simulink library "sm_backhoe_lib"  (R2021b)
settings: Solver=ode45  StartTime=0.0  StopTime=10.0  RelTol=1e-3  EnableMultiTasking=on
undefined symbols (not defined in the file): X, Y, Z
libraries: sm_lib x45, fl_lib x12, $bdroot x7, nesl_utility x4, simulink x1
(part 1 of 2)
settings Model: Creator=The MathWorks, Inc.  LastModifiedBy=The MathWorks, Inc.
settings SolverCC: AlgebraicLoopSolver=TrustRegion
settings DataIOCC: LimitDataPoints=on  SaveFormat=Array  SignalLoggingSaveFormat=ModelDataLogs  ReturnWorkspaceOutputs=off
settings OptimizationCC: ExpressionDepthLimit=2147483647  LifeSpan=inf
settings DebuggingCC: UnderspecifiedInitializationDetection=Classic  MergeDetectMultiDrivingBlocksExec=none  SolverPrmCheckMsg=warning  MultiTaskDSMMsg=warning  MultiTaskCondExecSysMsg=none  StateNameClashWarn=warning  SFUnexpectedBacktrackingDiag=warning  SFNoUnconditionalDefaultTransitionDiag=warning  SFExecutionAtInitializationDiag=none  SFMachineParentedDataDiag=warning  ArithmeticOperatorsInVariantConditions=warning
settings HardwareCC: ProdBitPerPointer=32  ProdBitPerSizeT=32  ProdBitPerPtrDiffT=32  ProdLargestAtomicFloat=None  ProdIntDivRoundTo=Undefined  ProdEndianess=Unspecified  ProdWordSize=32  ProdHWDeviceType=32-bit Generic
settings ModelReferenceCC: PropagateSignalLabelsOutOfModel=off
settings SFSimCC: SimUseLocalCustomCode=off  CustomCodeUndefinedFunction=UseInterfaceOnly
settings RTWCC: RTWUseLocalCustomCode=off
settings CodeAppCC: StateflowObjectComments=on
settings GRTTargetCC: TargetLangStandard=C89/C90 (ANSI)
settings ConfigComp: CovMetricSettings=dw  CovSaveCumulativeToWorkspaceVar=on  CovSaveSingleToWorkspaceVar=on  CovExternalEMLEnable=off

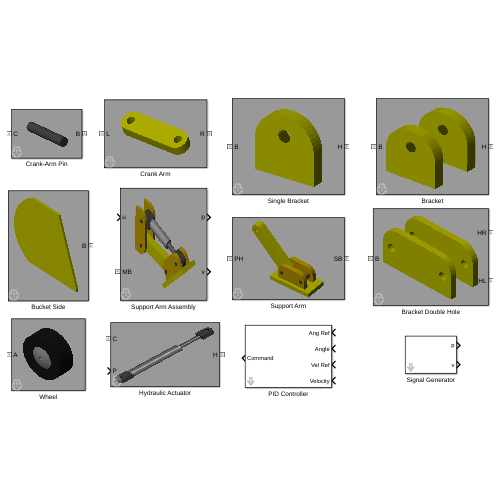
[thumbnail: Simulink's stored preview of the top-level diagram]
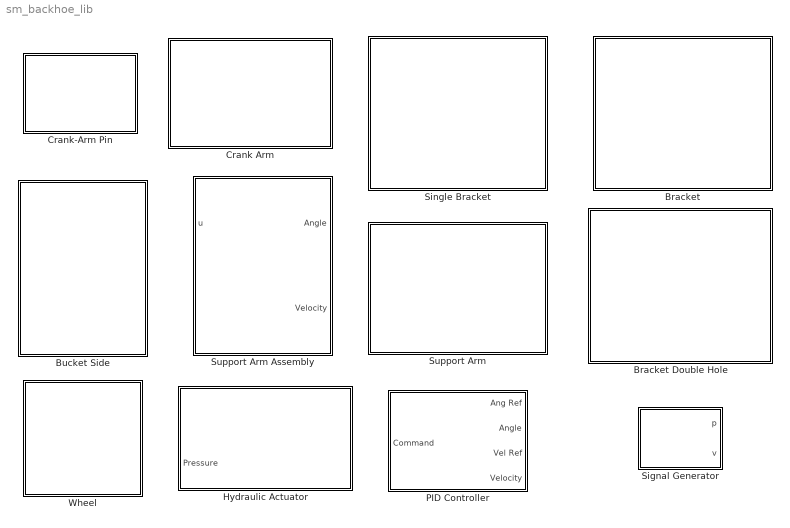
== system sm_backhoe_lib ==
  Bracket : Subsystem  mask(Bracket){Hbracket=0.75, Wbracket=0.75, Tbracket=0.15, Dbracket=0.8, Hhole=0.5, Rhole=0.075, circlePoints=25, bracketColor=[0.8 0.8 0], rho=7780}
      mask prompts: Hbracket "Hbracket (m)"; Wbracket "Wbracket (m)"; Tbracket "Tbracket (m)"; Dbracket "Dbracket (m)"; Hhole "Hhole (m)"; Rhole "Rhole (m)"; circlePoints "Circle Resolution (pts/rev)"; bracketColor "Bracket Color"; rho "Density (kg/m^3)"
      mask help:
      | Consists of the backhoe bracket assembly.
      |
      | Attachment points are:
      | B: The base of the bracket.
      | H: The center point between the two holes, which is configured for Revolute joints.
      |
      | Click on Help to view a schematic of the bracket, its configurable dimension parameters and attachment points (in red).
      mask init:
      | bracketPoints = [];
      | 
      | %% Bracket mold.
      | y = Hbracket - (Wbracket/2);
      | for i = 0:circlePoints
      |     angle = (i/circlePoints)*pi;
      |     bracketPoints = [bracketPoints; ...
      |                     (Wbracket/2)*cos(angle) (y+(Wbracket/2)*sin(angle))];
      | end
      | bracketPoints = [bracketPoints; ...
      |                  -Wbracket/2 0;0 0];
      |              
      | %% Hole
      | for i = 0:circlePoints*2
      |     angle = -pi/2 - (i/circlePoints)*pi;
      |     bracketPoints = [bracketPoints; ...
      |                     Rhole*cos(angle) (Hhole+(Rhole*sin(angle)))];
      | end
      | bracketPoints = [bracketPoints; ...
      |                  0 0;Wbracket/2 0];
      |                  
      | %% Uncomment to plot the cross-sections
      | % close all;
      | % figure;
      | % plot(bracketPoints(:,1),bracketPoints(:,2),'b*-');
      mask Help: web(fullfile(matlabroot,'toolbox','physmod','sm','smdemos','backhoe','demohelp','sm_backhoe_bracket.html'));
      mask Display:
      | image(fullfile(matlabroot,'toolbox','physmod','sm','smdemos','backhoe','images','sm_backhoe_bracket.png'));
      | port_label('lconn',1,'B');
      | port_label('rconn',1,'H');
  Bracket Double Hole : Subsystem  mask(Bracket Double Hole){Hbracket=1, Wbracket=2, Tbracket=0.15, Dbracket=0.8, Hhole=0.5, Dhole=1.5, Rhole=0.1, Rfillet=0.4, Nc=25, bracketColor=[0.8 0.8 0], rho=7780}
      mask prompts: Hbracket "Hbracket (m)"; Wbracket "Wbracket (m)"; Tbracket "Tbracket (m)"; Dbracket "Dbracket (m)"; Hhole "Hhole (m)"; Dhole "Dhole (m)"; Rhole "Rhole (m)"; Rfillet "Rfillet (m)"; Nc "Circle Resolution (pts/rev)"; bracketColor "Bracket Color"; rho "Density (kg/m^3)"
      mask help:
      | Consists of the backhoe double-hole bracket assembly.
      |
      | Attachment points are:
      | B: The base of the bracket.
      | HL: The center point between the two left holes, which is configured for Revolute joints.
      | HR: The center point between the two right holes, which is configured for Revolute joints.
      |
      | Click on Help to view a schematic of the bracket, its configurable dimension parameters and attachment points (in red).
      mask init:
      | %% Right Hole
      | bracketPoints = [0 0; Dhole/2 0];
      | angle = linspace(-pi/2,-5*pi/2,Nc)';
      | bracketPoints = [bracketPoints; ...
      |                  (Dhole/2+Rhole*cos(angle)) (Hhole+Rhole*sin(angle))];
      | bracketPoints = [bracketPoints; Dhole/2 0];                 
      | 
      | %% Bracket Outer Boundary
      | bracketPoints = [bracketPoints; Wbracket/2 0];
      | x = Wbracket/2 - Rfillet;
      | y = Hbracket - Rfillet;
      | angle = linspace(0,pi/2,Nc/4)';
      | bracketPoints = [bracketPoints; ...
      |                  (x+Rfillet*cos(angle)) (y+Rfillet*sin(angle))];
      | 
      | angle = linspace(pi/2,pi,Nc/4)';             
      | bracketPoints = [bracketPoints; ...
      |                  (-x+Rfillet*cos(angle)) (y+Rfillet*sin(angle))];
      | bracketPoints = [bracketPoints; -Wbracket/2 0];
      |                  
      | %% Left Hole
      | bracketPoints = [bracketPoints;-Dhole/2 0];
      | angle = linspace(-pi/2,-5*pi/2,Nc)';
      | bracketPoints = [bracketPoints; ...
      |                  (-Dhole/2+Rhole*cos(angle)) (Hhole+Rhole*sin(angle))];
      | bracketPoints = [bracketPoints;-Dhole/2 0];
      mask Help: web(fullfile(matlabroot,'toolbox','physmod','sm','smdemos','backhoe','demohelp','sm_backhoe_bracket2.html'));
      mask Display:
      | image(fullfile(matlabroot,'toolbox','physmod','sm','smdemos','backhoe','images','sm_backhoe_bracket2.png'));
      | port_label('lconn',1,'B');
      | port_label('rconn',1,'HR');
      | port_label('rconn',2,'HL');
  Bucket Side : Subsystem  mask(Bucket Side){bucketUpper=1.3, bucketLower=2, bucketHeight=2, bucketThickness=0.05, chordAngle=pi/6, Nc=45, color=[0.8 0.8 0], rho=7780}
      mask prompts: bucketUpper "Wupper (m)"; bucketLower "Wlower (m)"; bucketHeight "Hbucket (m)"; bucketThickness "Tbucket (m)"; chordAngle "alpha (radians)"; Nc "Circle Resolution (pts/rev)"; rho "Density (kg/m^3)"
      mask help:
      | Consists of the backhoe bucket side plate, which is used as an auxiliary library block inside the Bucket block.
      |
      | Click on Help to view a schematic of the bucket, its configurable dimension parameters and attachment points (in red).
      mask init:
      | bucketRadius = bucketHeight/(2*cos(chordAngle));
      | 
      | Nch = Nc*(pi-2*chordAngle)/(2*pi);
      | angle = linspace(-pi/2+chordAngle, pi/2-chordAngle,Nch)'; 
      | bucketSide = [(bucketRadius*cos(angle)-bucketRadius*sin(chordAngle)) ...
      |        bucketRadius*sin(angle)];
      | 
      | bucketSide = [ bucketSide; ...
      |               -bucketUpper bucketHeight/2; ...
      |               -bucketLower -(bucketHeight/2 - bucketThickness);...
      |               -bucketLower -bucketHeight/2];
      mask Help: web(fullfile(matlabroot,'toolbox','physmod','sm','smdemos','backhoe','demohelp','sm_backhoe_bucket.html'));
      mask Display:
      | image(fullfile(matlabroot,'toolbox','physmod','sm','smdemos','backhoe','images','sm_backhoe_bucketside.png'));
      | port_label('rconn',1,'B');
  Crank Arm : Subsystem  mask(Crank Arm){L=1, W=0.25, T=0.1, D=0.75, R=0.05, Nc=25, color=[0.8 0.8 0], rho=7780}
      mask prompts: L "L (m)"; W "W (m)"; T "T (m)"; D "D (m)"; R "Rhole (m)"; Nc "Circle Resolution (pts/rev)"; rho "Density (kg/m^3)"
      mask help:
      | Parameterized bar with rounded ends and two holes for attachment.
      |
      | Attachment points are the left (L) and right (R) holes of the crank arm, which are configured for Revolute Joints.
      |
      | Click on Help to view a schematic of the bracket, its configurable dimension parameters and attachment points (in red).
      mask init:
      | crankPoints = [];
      | 
      | % Crank 1
      | x = (L - W)/2;
      | angle = linspace(-pi/2,pi/2,Nc/2)';
      | crankPoints = [crankPoints; ...
      |       (x + W*cos(angle)/2) W*sin(angle)/2];
      |   
      | x = D/2;
      | angle = linspace(pi/2,-3*pi/2,Nc)';
      | crankPoints = [crankPoints; ...
      |       (x + R*cos(angle)) R*sin(angle)];
      | 
      | crankPoints = [crankPoints;x W/2];
      | x = -D/2;
      | crankPoints = [crankPoints;x W/2];
      | 
      | angle = linspace(pi/2,-3*pi/2,Nc)';
      | crankPoints = [crankPoints; ...
      |       (x + R*cos(angle)) R*sin(angle)];
      | 
      | x = -(L - W)/2;
      | angle = linspace(pi/2,3*pi/2,Nc/2)';
      | crankPoints = [crankPoints; ...
      |       (x + W*cos(angle)/2) W*sin(angle)/2];
      mask Help: web(fullfile(matlabroot,'toolbox','physmod','sm','smdemos','backhoe','demohelp','sm_backhoe_crankarm.html'));
      mask DialogControl ParameterTabVar0 Prompt: Geometry
      mask DialogControl ParameterTabVar01 Prompt: Material Properties
      mask Display:
      | image(fullfile(matlabroot,'toolbox','physmod','sm','smdemos','backhoe','images','sm_backhoe_crankarm.png'));
      | port_label('lconn',1,'L');
      | port_label('rconn',1,'R');
  Crank-Arm Pin : Subsystem  mask(Crank-Arm Pin){R=0.1, L=1, T=0.1, color=[0.3 0.3 0.3], rho=7780}
      mask prompts: R "Radius (m)"; L "Length (m)"; T "Crank Arm Thickness (m)"; rho "Density (kg/m^3)"
      mask help:
      | Parameterized block for the two pins that extrude from the Upper Arm. These pins connect to the crank arms, which create a four-bar linkage with the Upper Arm and the Bucket.
      |
      | Attachment points are:
      | B: Base of the pin.
      | C: Crank arm attachment point which is configured for Revolute joints.
      mask Display:
      | image(repmat(imread(fullfile(matlabroot,'toolbox','physmod','sm','smdemos','backhoe','images','sm_backhoe_crankpin.png')),[1 1 3]));
      | port_label('lconn',1,'C');
      | port_label('rconn',1,'B');
  Hydraulic Actuator : Subsystem  mask(Hydraulic Actuator){Lcyl=2.5, Rcyl=0.2, Lbase=0.65, Wbase=0.35, Rbp=0.075, Lbp=0.8, circlePointsCyl=25, circlePointsCylB=25, Lpist=2.5, Rpist=0.1, Whead=0.35, Lhead=0.65, Rhp=0.075, Lhp=0.9, circlePointsPist=25, cylColor=[0.6 0.6 0.6], rhoCyl=7780, pistColor=[0.4 0.4 0.4], rhoPist=7780, connColor=[0.3 0.3 0.3], rhoConn=7780}
      mask prompts: Lcyl "Lcyl (m)"; Rcyl "Rcyl (m)"; Lbase "Lbase (m)"; Wbase "Wbase(m)"; Rbp "Rbp (m)"; Lbp "Lbp (m)"; circlePointsCyl "Circle Resolution (pts/rev)"; circlePointsCylB "Bracket Circle Resolution (pts/rev)"; Lpist "Lpist (m)"; Rpist "Rpist (m)"; Whead "Whead (m)"; Lhead "Lhead (m)"; Rhp "Rhp (m)"; Lhp "Lhp (m)"; circlePointsPist "Bracket Circle Resolution (pts/rev)"; cylColor "Cylinder Color"; rhoCyl "Cylinder Density (kg/m^3)"; pistColor "Piston Color"; rhoPist "Piston Density (kg/m^3)"; connColor "Connector Color"; rhoConn "Connector Density (kg/m^3)"
      mask help:
      | Consists of the backhoe hydraulic actuator assembly.
      |
      | Zero piston displacement corresponds to the piston and cylinder centers of mass in the same position. Positive piston displacement is outward motion, and negative piston displacement is inward motion.
      |
      | Attachment points are:
      | C: Center of the Cylinder base bracket hole.
      | H: Center of the Piston Head bracket hole.
      | Both attachment points are configured for Revolute joints.
      |
      | The Simulink Signal input port supplies a Pressure value P (in bar) to a Simscape hydraulic network.
      |
      | Click on Help to view a schematic of the hydraulic actuator, its configurable dimension parameters and attachment points (in red).
      mask init:
      | % Hollow Cylinder cross-section
      | angles = (0:circlePointsCyl)' * 2 * pi / circlePointsCyl;
      | unit_circle = [cos(angles) sin(angles)];
      | unit_circle_cw = flipud(unit_circle);
      | cylSection = [Rcyl * unit_circle; Rpist * unit_circle_cw];
      mask Help: web(fullfile(matlabroot,'toolbox','physmod','sm','smdemos','backhoe','demohelp','sm_backhoe_actuator.html'));
      mask DialogControl ParameterTabVar0 Prompt: Cylinder
      mask DialogControl ParameterTabVar01 Prompt: Piston
      mask DialogControl ParameterTabVar012 Prompt: Material Properties
      mask Display:
      | image(repmat(imread(fullfile(matlabroot,'toolbox','physmod','sm','smdemos','backhoe','images','sm_backhoe_actuator.png')),[1 1 3]));
      | port_label('rconn',1,'H');
      | port_label('lconn',1,'C');
      | port_label('input',1,'P');
  PID Controller : Subsystem  mask(PID Controller){upperLim=-40, lowerLim=-100, Kp=40, Ki=1, Kd=2}
      mask prompts: upperLim "Upper Limit (deg)"; lowerLim "Lower Limit (deg)"; Kp "Proportional Gain, Kp"; Ki "Integral Gain, Ki"; Kd "Derivative Gain, Kd"
      mask help: This block takes in a reference angle and measured angle, and uses a PID Controller with saturation to give a control command.
  Signal Generator : Subsystem  mask(Signal Generator){T=[0 10 20 30 40 50 60], P=[0 1 1 0 0 1 -1]}
      mask prompts: T "Time values (sec)"; P "Position values (sec)"
      mask help: The block outputs the position and velocity signals given the piece-wise linear position signal. The input time values have to be monotonically increasing (no repetitions).
      mask init:
      | Tdiff = diff(T);
      | Pdiff = diff(P);
      | v = Pdiff./Tdiff;
      | 
      | if(any(Tdiff <= 0))
      |     errordlg('Time values have to be monotonically increasing (no repetitions)');
      | end
      | V = zeros(2*length(v),1);
      | V(1:2:2*length(v)) = v;
      | V(2:2:2*length(v)) = v;
      | 
      | Tv = zeros(2*length(v),1);
      | Tv(1) = T(1); Tv(end) = T(end);
      | Tv(2:2:end-1) = T(2:end-1)-0.01;
      | Tv(3:2:end-1) = T(2:end-1)+0.01;
  Single Bracket : Subsystem  mask(Single Bracket){Hbracket=0.75, Wbracket=0.75, Tbracket=0.15, Hhole=0.5, Rhole=0.075, Nc=25, bracketColor=[0.8 0.8 0], rho=7780}
      mask prompts: Hbracket "Hbracket (m)"; Wbracket "Wbracket (m)"; Tbracket "Tbracket (m)"; Hhole "Hhole (m)"; Rhole "Rhole (m)"; Nc "Circle Resolution (pts/rev)"; bracketColor "Bracket Color"; rho "Density (kg/m^3)"
      mask help:
      | Consists of the backhoe single bracket assembly.
      |
      | Attachment points are:
      | B: The base of the bracket.
      | H: The center point of the hole, which is configured for Revolute joints.
      |
      | Click on Help to view a schematic of the bracket, its configurable dimension parameters and attachment points (in red).
      mask init:
      | bracketPoints = [];
      | 
      | %% Bracket mold.
      | y = Hbracket - (Wbracket/2);
      | angle = linspace(0,pi,Nc/2)';
      | bracketPoints = [(Wbracket/2)*cos(angle) (y+(Wbracket/2)*sin(angle))];
      | bracketPoints = [bracketPoints; ...
      |                  -Wbracket/2 0;0 0];
      |              
      | %% Hole
      | angle = linspace(3*pi/2,-pi/2,Nc)';
      | bracketPoints = [bracketPoints; ...
      |                  Rhole*cos(angle) (Hhole+(Rhole*sin(angle)))];
      | bracketPoints = [bracketPoints; ...
      |                  0 0;Wbracket/2 0];
      mask Help: web(fullfile(matlabroot,'toolbox','physmod','sm','smdemos','backhoe','demohelp','sm_backhoe_singlebracket.html'));
      mask Display:
      | image(fullfile(matlabroot,'toolbox','physmod','sm','smdemos','backhoe','images','sm_backhoe_bracket1.png'));
      | port_label('lconn',1,'B');
      | port_label('rconn',1,'H');
  Support Arm : Subsystem  mask(Support Arm){Larm=2.5, Warm=0.5, Tarm=0.35, Dhole=2, Rhole=0.075, initAngle=45, Lpin=0.8, circlePointsArm=25, Lfoot=2, Wfoot=1, Tfoot=0.2, Dconn=1, Hhole=0.3, Rfillet=0.4, circlePointsFoot=25, armColor=[0.8 0.8 0], bracketColor=[0.8 0.65 0], footColor=[0.8 0.8 0], pinColor=[0.3 0.3 0.3], rho=7780}
      mask prompts: Larm "Larm (m)"; Warm "Warm (m)"; Tarm "Tarm (m)"; Dhole "Dhole (m)"; Rhole "Rhole (m)"; initAngle "Initial Arm-Foot Angle (deg)"; Lpin "Lpin (m)"; circlePointsArm "Circle Resolution (pts/rev)"; Lfoot "Lfoot (m)"; Wfoot "Wfoot (m)"; Tfoot "Tfoot (m)"; Dconn "Dconn (m)"; Hhole "Hhole (m)"; Rfillet "Rfillet (m)"; circlePointsFoot "Circle Resolution (pts/rev)"; armColor "Arm Color"; bracketColor "Bracket Color"; footColor "Foot Color"; pinColor "Pin Color"; rho "Density (kg/m^3)"
      mask help:
      | Consists of the backhoe support arm that connects an arm, a bracket and a foot.
      |
      | Attachment points are:
      | SB: The free hole of the crank arm, which connects to the Shoulder Bracket.
      | PH: The free pin of the foot bracket, which connect to the piston head of a hydraulic actuator.
      | Both attachment points are configured for Revolute Joints.
      |
      | Click on Help to view a schematic of the support arm, its configurable dimension parameters and attachment points (in red).
      mask Help: web(fullfile(matlabroot,'toolbox','physmod','sm','smdemos','backhoe','demohelp','sm_backhoe_supportarm.html'));
      mask Display:
      | image(fullfile(matlabroot,'toolbox','physmod','sm','smdemos','backhoe','images','sm_backhoe_supportarm.png'));
      | port_label('lconn',1,'PH');
      | port_label('rconn',1,'SB');
  Support Arm Assembly : Subsystem  mask(Support Arm Assembly){Hbracket=0.8, Wbracket=1.75, Tbracket=0.15, Dbracket=0.8, HShoulderHole=0.5, DShoulderHole=1, RShoulderHole=0.075, RShoulderFillet=0.4, Larm=2.5, Warm=0.5, Tarm=0.35, Dhole=2, Rhole=0.075, AFAngle=45, Lpin=0.85, Lfoot=2, Wfoot=1, Tfoot=0.2, Dconn=1, Hhole=0.3, Rfillet=0.4, Lcyl=1.35, Rcyl=0.2, Lbase=0.65, Wbase=0.425, Rbp=0.075, Lbp=0.8, Lpist=1.35, Rpist=0.1, Lhead=0.5, Whead=0.275, Rhp=0.075, Lhp=0.8, circlePointsPist=25, circlePointsCyl=25, circlePointsCylB=25, circlePointsShoulder=25, circlePointsArm=25, circlePointsFoot=25, shoulderColor=[1 0.6 0], armColor=[1 0.8 0], bracketColor=[1 0.6 0], footColor=[1 0.8 0], pinColor=[0.5 0.5 0.5], pistonGray=[0.4 0.4 0.4], cylinderGray=[0.6 0.6 0.6], rho=7780}
      mask prompts: Hbracket "Hbracket (m)"; Wbracket "Wbracket (m)"; Tbracket "Tbracket (m)"; Dbracket "Dbracket (m)"; HShoulderHole "HShoulderHole (m)"; DShoulderHole "DShoulderHole (m)"; RShoulderHole "RShoulderHole (m)"; RShoulderFillet "RShoulderFillet (m)"; Larm "Larm (m)"; Warm "Warm (m)"; Tarm "Tarm (m)"; Dhole "Dhole (m)"; Rhole "Rhole (m)"; AFAngle "Arm-Foot Angle (deg)"; Lpin "Lpin (m)"; Lfoot "Lfoot (m)"; Wfoot "Wfoot (m)"; Tfoot "Tfoot (m)"; Dconn "Dconn (m)"; Hhole "Hhole (m)"; Rfillet "Rfillet (m)"; Lcyl "Lcyl (m)"; Rcyl "Rcyl (m)"; Lbase "Lbase (m)"; Wbase "Wbase (m)"; Rbp "Rbp (m)"; Lbp "Lbp (m)"; Lpist "Lpist (m)"; Rpist "Rpist (m)"; Lhead "Lhead (m)"; Whead "Whead (m)"; Rhp "Rhp (m)"; Lhp "Lhp (m)"; circlePointsPist "Bracket Circle Resolution (pts/rev)"; circlePointsCyl "Circle Resolution (pts/rev)"; circlePointsCylB "Bracket Circle Resolution (pts/rev)"; circlePointsShoulder "Circle Resolution (pts/rev)"; circlePointsArm "Circle Resolution (pts/rev)"; circlePointsFoot "Circle Resolution (pts/rev)"; shoulderColor "Shoulder Bracket Color"; armColor "Arm Color"; bracketColor "Foot Bracket Color"; footColor "Foot Color"; pinColor "Pin Color"; pistonGray "Piston Color"; cylinderGray "Cylinder Color"; rho "Density (kg/m^3)"
      mask help:
      | Consists of a backhoe support arm, a shoulder bracket and a hydraulic actuator.
      |
      | Attachment points are:
      | MB: The base of the shoulder bracket, which connects rigidly to the Mounting Base.
      |
      | Inputs and outputs are:
      | u: The pressure to the hydraulic actuator.
      | a: The angle of the support arm, for sensing.
      |
      | Click on Help to view a schematic of the support arm assembly, its configurable dimension parameters and attachment points (in red).
      mask Help: web(fullfile(matlabroot,'toolbox','physmod','sm','smdemos','backhoe','demohelp','sm_backhoe_supportassembly.html'));
      mask Display:
      | image(fullfile(matlabroot,'toolbox','physmod','sm','smdemos','backhoe','images','sm_backhoe_supportassembly.png'));
      | port_label('input',1,'u');
      | port_label('output',1,'p');
      | port_label('output',2,'v');
      | port_label('lconn',1,'MB');
  Wheel : Subsystem  mask(Wheel){Rwheel=0.5, Rtire=1, Raxle=0.075, W=0.75, Nc=30, tireColor=[0.1 0.1 0.1], rhoTire=1500, wheelColor=[0.6 0.6 0.6], rhoWheel=7780}
      mask prompts: Rwheel "Wheel Radius (m)"; Rtire "Tire Radius (m)"; Raxle "Axle Radius (m)"; W "Wheel Width (m)"; Nc "Circle Resolution (pts/rev)"; tireColor "Tire Color"; rhoTire "Tire Density (kg/m^3)"; wheelColor "Wheel Color"; rhoWheel "Wheel Density (kg/m^3)"
      mask help:
      | Consists of the backhoe wheel assembly.
      |
      | Attachment points are:
      | A: The center of the wheel's axle.
      mask init:
      | % Circles
      | angles = (0:Nc)' * 2 * pi / Nc;
      | unit_circle = [cos(angles) sin(angles)];
      | unit_circle_cw = flipud(unit_circle);
      | 
      | % Wheel
      | wheelPoints = [Rwheel * unit_circle; Raxle * unit_circle_cw];
      | 
      | % Tire
      | tirePoints = [Rtire * unit_circle; Rwheel * unit_circle_cw];
      | 
      | % Rim
      | H = W*0.15;
      | k = H/(Rwheel^2);
      | vec = linspace(Rwheel,Raxle,10)';
      | rimPoints = [Raxle 0; vec  H-k*vec.^2];
      mask Display:
      | image(repmat(imread(fullfile(matlabroot,'toolbox','physmod','sm','smdemos','backhoe','images','sm_backhoe_wheel.png')),[1 1 3]));
      | port_label('lconn',1,'A');

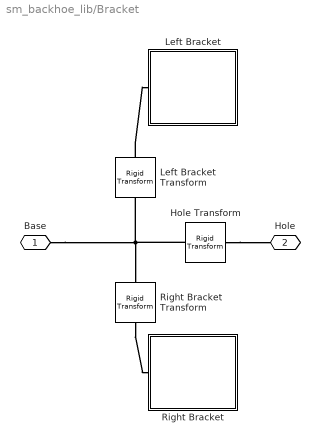
== system sm_backhoe_lib/Bracket ==
  Hole Transform : sm_lib/Frames and Transforms/Rigid Transform  TranslationMethod=StandardAxis  TranslationStandardOffset=Hhole  TranslationLengthUnit=m  TranslationStandardAxis=+Z  TranslationCartesianOffset=[-(Dbracket-Tbracket)/2 0 Hhole]  TranslationROffset=0  TranslationROffsetUnits=m  TranslationZOffset=0  TranslationZOffsetUnits=m  TranslationThetaOffset=0  TranslationThetaOffsetUnits=deg  RotationMethod=AlignedAxes  RotationAngleUnits=deg  RotationStandardAxis=+X  RotationAngle=90  RotationArbitraryAxis=[0 0 1]  FollAlignAxisA=+Z  BaseAlignAxisA=-Y  FollAlignAxisB=+X  BaseAlignAxisB=+X  RotationSequenceAxes=FollowerAxes  RotationSequence=XYX  RotationSequenceAngles=[0 0 0]  RotationSequenceAnglesUnits=deg  RotationMatrix=[1 0 0; 0 1 0; 0 0 1]
  Left Bracket : Subsystem  mask(Single Bracket){Hbracket=Hbracket, Wbracket=Wbracket, Tbracket=Tbracket, Hhole=Hhole, Rhole=Rhole, Nc=circlePoints, bracketColor=bracketColor, rho=rho}
      mask prompts: Hbracket "Hbracket (m)"; Wbracket "Wbracket (m)"; Tbracket "Tbracket (m)"; Hhole "Hhole (m)"; Rhole "Rhole (m)"; Nc "Circle Resolution (pts/rev)"; bracketColor "Bracket Color"; rho "Density (kg/m^3)"
      mask help:
      | Consists of the backhoe single bracket assembly.
      |
      | Attachment points are:
      | B: The base of the bracket.
      | H: The center point of the hole, which is configured for Revolute joints.
      |
      | Click on Help to view a schematic of the bracket, its configurable dimension parameters and attachment points (in red).
      mask init: same as sm_backhoe_lib/Single Bracket
      mask Help: web(fullfile(matlabroot,'toolbox','physmod','sm','smdemos','backhoe','demohelp','sm_backhoe_singlebracket.html'));
      mask Display:
      | image(fullfile(matlabroot,'toolbox','physmod','sm','smdemos','backhoe','images','sm_backhoe_bracket1.png'));
      | port_label('lconn',1,'B');
  Left Bracket Transform : sm_lib/Frames and Transforms/Rigid Transform  TranslationMethod=StandardAxis  TranslationStandardOffset=(Dbracket-Tbracket)/2  TranslationLengthUnit=m  TranslationStandardAxis=-Y  TranslationCartesianOffset=[0 0 0]  TranslationROffset=0  TranslationROffsetUnits=m  TranslationZOffset=0  TranslationZOffsetUnits=m  TranslationThetaOffset=0  TranslationThetaOffsetUnits=deg  RotationMethod=None  RotationAngleUnits=deg  RotationStandardAxis=+X  RotationAngle=90  RotationArbitraryAxis=[0 0 1]  FollAlignAxisA=+X  BaseAlignAxisA=+X  FollAlignAxisB=+Y  BaseAlignAxisB=+Z  RotationSequenceAxes=FollowerAxes  RotationSequence=XYX  RotationSequenceAngles=[0 0 0]  RotationSequenceAnglesUnits=deg  RotationMatrix=[1 0 0; 0 1 0; 0 0 1]
  Right Bracket : Subsystem  mask(Single Bracket){Hbracket=Hbracket, Wbracket=Wbracket, Tbracket=Tbracket, Hhole=Hhole, Rhole=Rhole, Nc=circlePoints, bracketColor=bracketColor, rho=rho}
      mask prompts: Hbracket "Hbracket (m)"; Wbracket "Wbracket (m)"; Tbracket "Tbracket (m)"; Hhole "Hhole (m)"; Rhole "Rhole (m)"; Nc "Circle Resolution (pts/rev)"; bracketColor "Bracket Color"; rho "Density (kg/m^3)"
      mask help:
      | Consists of the backhoe single bracket assembly.
      |
      | Attachment points are:
      | B: The base of the bracket.
      | H: The center point of the hole, which is configured for Revolute joints.
      |
      | Click on Help to view a schematic of the bracket, its configurable dimension parameters and attachment points (in red).
      mask init: same as sm_backhoe_lib/Single Bracket
      mask Help: web(fullfile(matlabroot,'toolbox','physmod','sm','smdemos','backhoe','demohelp','sm_backhoe_singlebracket.html'));
      mask Display:
      | image(fullfile(matlabroot,'toolbox','physmod','sm','smdemos','backhoe','images','sm_backhoe_bracket1.png'));
      | port_label('lconn',1,'B');
  Right Bracket Transform : sm_lib/Frames and Transforms/Rigid Transform  TranslationMethod=StandardAxis  TranslationStandardOffset=(Dbracket-Tbracket)/2  TranslationLengthUnit=m  TranslationStandardAxis=+Y  TranslationCartesianOffset=[0 (Dbracket-Tbracket)/2 Hbracket/2]  TranslationROffset=0  TranslationROffsetUnits=m  TranslationZOffset=0  TranslationZOffsetUnits=m  TranslationThetaOffset=0  TranslationThetaOffsetUnits=deg  RotationMethod=None  RotationAngleUnits=deg  RotationStandardAxis=+X  RotationAngle=90  RotationArbitraryAxis=[0 0 1]  FollAlignAxisA=+X  BaseAlignAxisA=+X  FollAlignAxisB=+Y  BaseAlignAxisB=+Z  RotationSequenceAxes=FollowerAxes  RotationSequence=XYX  RotationSequenceAngles=[0 0 0]  RotationSequenceAnglesUnits=deg  RotationMatrix=[1 0 0; 0 1 0; 0 0 1]
  Base : PMIOPort  Side=Left
  Hole : PMIOPort  Port=2  Side=Right
  connections:
  Base/RConn1 -- Hole Transform/LConn1 -- Left Bracket Transform/LConn1 -- Right Bracket Transform/LConn1
  Right Bracket Transform/RConn1 -- Right Bracket/LConn1
  Left Bracket Transform/RConn1 -- Left Bracket/LConn1
  Hole Transform/RConn1 -- Hole/RConn1

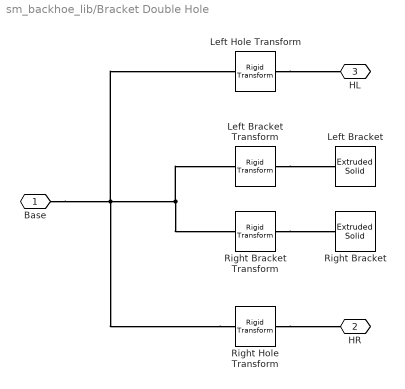
== system sm_backhoe_lib/Bracket Double Hole ==
  Left Bracket : sm_lib/Body Elements/Extruded Solid  GraphicAmbientColor=[0.15 0.15 0.15 1.0]  BasedOnType=Density  CenterOfMass=[0 0 0]  CenterOfMassUnits=m  GraphicDiffuseColor=bracketColor  ExportConvexHullGeometry=off  ExtrusionCrossSection=bracketPoints  ExtrusionCrossSectionUnits=m  Density=rho  DensityUnits=kg/(m^3)  DoExposeReferenceFrame=on  GraphicEmissiveColor=[0.0 0.0 0.0 1.0]  ExportEntireGeometry=off  ExtrusionLength=Tbracket  ExtrusionLengthUnits=m  ExtrusionType=General  SerializedFrames=<Frames/>  MarkerShape=Sphere  MarkerSize=10  GraphicType=FromGeometry  InertiaType=CalculateFromGeometry  Mass=1  MassUnits=kg  MomentsOfInertia=[1 1 1]  MomentsOfInertiaUnits=kg*m^2  PolygonNumSides=3  GraphicOpacity=1.0  PolygonOuterRadius=1  PolygonOuterRadiusUnits=m  ProductsOfInertia=[0 0 0]  ProductsOfInertiaUnits=kg*m^2  GraphicShininess=75  GraphicSpecularColor=[0.5 0.5 0.5 1.0]  GraphicVisPropType=SimpleVisualProperties
  Left Bracket Transform : sm_lib/Frames and Transforms/Rigid Transform  TranslationMethod=StandardAxis  TranslationStandardOffset=(Dbracket-Tbracket)/2  TranslationLengthUnit=m  TranslationStandardAxis=-Y  TranslationCartesianOffset=[0 0 0]  TranslationROffset=0  TranslationROffsetUnits=m  TranslationZOffset=0  TranslationZOffsetUnits=m  TranslationThetaOffset=0  TranslationThetaOffsetUnits=deg  RotationMethod=AlignedAxes  RotationAngleUnits=deg  RotationStandardAxis=+X  RotationAngle=90  RotationArbitraryAxis=[0 0 1]  FollAlignAxisA=+X  BaseAlignAxisA=+X  FollAlignAxisB=+Y  BaseAlignAxisB=+Z  RotationSequenceAxes=FollowerAxes  RotationSequence=XYX  RotationSequenceAngles=[0 0 0]  RotationSequenceAnglesUnits=deg  RotationMatrix=[1 0 0; 0 1 0; 0 0 1]
  Left Hole Transform : sm_lib/Frames and Transforms/Rigid Transform  TranslationMethod=Cartesian  TranslationStandardOffset=Hhole  TranslationLengthUnit=m  TranslationStandardAxis=+Z  TranslationCartesianOffset=[-Dhole/2 0 Hhole]  TranslationROffset=0  TranslationROffsetUnits=m  TranslationZOffset=0  TranslationZOffsetUnits=m  TranslationThetaOffset=0  TranslationThetaOffsetUnits=deg  RotationMethod=AlignedAxes  RotationAngleUnits=deg  RotationStandardAxis=+X  RotationAngle=90  RotationArbitraryAxis=[0 0 1]  FollAlignAxisA=+X  BaseAlignAxisA=+X  FollAlignAxisB=+Y  BaseAlignAxisB=+Z  RotationSequenceAxes=FollowerAxes  RotationSequence=XYX  RotationSequenceAngles=[0 0 0]  RotationSequenceAnglesUnits=deg  RotationMatrix=[1 0 0; 0 1 0; 0 0 1]
  Right Bracket : sm_lib/Body Elements/Extruded Solid  GraphicAmbientColor=[0.15 0.15 0.15 1.0]  BasedOnType=Density  CenterOfMass=[0 0 0]  CenterOfMassUnits=m  GraphicDiffuseColor=bracketColor  ExportConvexHullGeometry=off  ExtrusionCrossSection=bracketPoints  ExtrusionCrossSectionUnits=m  Density=rho  DensityUnits=kg/(m^3)  DoExposeReferenceFrame=on  GraphicEmissiveColor=[0.0 0.0 0.0 1.0]  ExportEntireGeometry=off  ExtrusionLength=Tbracket  ExtrusionLengthUnits=m  ExtrusionType=General  SerializedFrames=<Frames/>  MarkerShape=Sphere  MarkerSize=10  GraphicType=FromGeometry  InertiaType=CalculateFromGeometry  Mass=1  MassUnits=kg  MomentsOfInertia=[1 1 1]  MomentsOfInertiaUnits=kg*m^2  PolygonNumSides=3  GraphicOpacity=1.0  PolygonOuterRadius=1  PolygonOuterRadiusUnits=m  ProductsOfInertia=[0 0 0]  ProductsOfInertiaUnits=kg*m^2  GraphicShininess=75  GraphicSpecularColor=[0.5 0.5 0.5 1.0]  GraphicVisPropType=SimpleVisualProperties
  Right Bracket Transform : sm_lib/Frames and Transforms/Rigid Transform  TranslationMethod=StandardAxis  TranslationStandardOffset=(Dbracket-Tbracket)/2  TranslationLengthUnit=m  TranslationStandardAxis=+Y  TranslationCartesianOffset=[0 (Dbracket-Tbracket)/2 Hbracket/2]  TranslationROffset=0  TranslationROffsetUnits=m  TranslationZOffset=0  TranslationZOffsetUnits=m  TranslationThetaOffset=0  TranslationThetaOffsetUnits=deg  RotationMethod=AlignedAxes  RotationAngleUnits=deg  RotationStandardAxis=+X  RotationAngle=90  RotationArbitraryAxis=[0 0 1]  FollAlignAxisA=+X  BaseAlignAxisA=+X  FollAlignAxisB=+Y  BaseAlignAxisB=+Z  RotationSequenceAxes=FollowerAxes  RotationSequence=XYX  RotationSequenceAngles=[0 0 0]  RotationSequenceAnglesUnits=deg  RotationMatrix=[1 0 0; 0 1 0; 0 0 1]
  Right Hole Transform : sm_lib/Frames and Transforms/Rigid Transform  TranslationMethod=Cartesian  TranslationStandardOffset=Hhole  TranslationLengthUnit=m  TranslationStandardAxis=+Z  TranslationCartesianOffset=[Dhole/2 0 Hhole]  TranslationROffset=0  TranslationROffsetUnits=m  TranslationZOffset=0  TranslationZOffsetUnits=m  TranslationThetaOffset=0  TranslationThetaOffsetUnits=deg  RotationMethod=AlignedAxes  RotationAngleUnits=deg  RotationStandardAxis=+X  RotationAngle=90  RotationArbitraryAxis=[0 0 1]  FollAlignAxisA=+X  BaseAlignAxisA=+X  FollAlignAxisB=+Y  BaseAlignAxisB=+Z  RotationSequenceAxes=FollowerAxes  RotationSequence=XYX  RotationSequenceAngles=[0 0 0]  RotationSequenceAnglesUnits=deg  RotationMatrix=[1 0 0; 0 1 0; 0 0 1]
  Base : PMIOPort  Side=Left
  HR : PMIOPort  Port=2  Side=Right
  HL : PMIOPort  Port=3  Side=Right
  connections:
  Right Hole Transform/RConn1 -- HR/RConn1
  Right Bracket Transform/RConn1 -- Right Bracket/RConn1
  Right Hole Transform/LConn1 -- Left Hole Transform/LConn1 -- Base/RConn1 -- Left Bracket Transform/LConn1 -- Right Bracket Transform/LConn1
  Left Bracket Transform/RConn1 -- Left Bracket/RConn1
  Left Hole Transform/RConn1 -- HL/RConn1

== system sm_backhoe_lib/Bucket Side ==
  Bucket Side : sm_lib/Body Elements/Extruded Solid  GraphicAmbientColor=[0.15 0.15 0.15 1.0]  BasedOnType=Density  CenterOfMass=[0 0 0]  CenterOfMassUnits=m  GraphicDiffuseColor=bucketColor  ExportConvexHullGeometry=off  ExtrusionCrossSection=bucketSide  ExtrusionCrossSectionUnits=m  Density=rhoSteel  DensityUnits=kg/(m^3)  DoExposeReferenceFrame=on  GraphicEmissiveColor=[0.0 0.0 0.0 1.0]  ExportEntireGeometry=off  ExtrusionLength=bucketThickness  ExtrusionLengthUnits=m  ExtrusionType=General  SerializedFrames=<Frames/>  MarkerShape=Sphere  MarkerSize=10  GraphicType=FromGeometry  InertiaType=CalculateFromGeometry  Mass=1  MassUnits=kg  MomentsOfInertia=[1 1 1]  MomentsOfInertiaUnits=kg*m^2  PolygonNumSides=3  GraphicOpacity=1.0  PolygonOuterRadius=1  PolygonOuterRadiusUnits=m  ProductsOfInertia=[0 0 0]  ProductsOfInertiaUnits=kg*m^2  GraphicShininess=75  GraphicSpecularColor=[0.5 0.5 0.5 1.0]  GraphicVisPropType=SimpleVisualProperties
  Bucket : PMIOPort  Side=Right
  connections:
  Bucket Side/RConn1 -- Bucket/RConn1

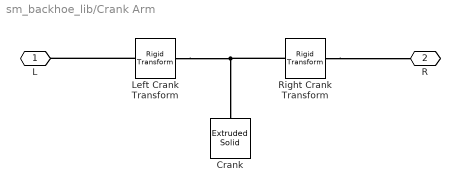
== system sm_backhoe_lib/Crank Arm ==
  Crank : sm_lib/Body Elements/Extruded Solid  GraphicAmbientColor=[0.15 0.15 0.15 1.0]  BasedOnType=Density  CenterOfMass=[0 0 0]  CenterOfMassUnits=m  GraphicDiffuseColor=color  ExportConvexHullGeometry=off  ExtrusionCrossSection=crankPoints  ExtrusionCrossSectionUnits=m  Density=rho  DensityUnits=kg/(m^3)  DoExposeReferenceFrame=on  GraphicEmissiveColor=[0.0 0.0 0.0 1.0]  ExportEntireGeometry=off  ExtrusionLength=T  ExtrusionLengthUnits=m  ExtrusionType=General  SerializedFrames=<Frames/>  MarkerShape=Sphere  MarkerSize=10  GraphicType=FromGeometry  InertiaType=CalculateFromGeometry  Mass=1  MassUnits=kg  MomentsOfInertia=[1 1 1]  MomentsOfInertiaUnits=kg*m^2  PolygonNumSides=3  GraphicOpacity=1.0  PolygonOuterRadius=1  PolygonOuterRadiusUnits=m  ProductsOfInertia=[0 0 0]  ProductsOfInertiaUnits=kg*m^2  GraphicShininess=75  GraphicSpecularColor=[0.5 0.5 0.5 1.0]  GraphicVisPropType=SimpleVisualProperties
  Left Crank Transform : sm_lib/Frames and Transforms/Rigid Transform  TranslationMethod=StandardAxis  TranslationStandardOffset=D/2  TranslationLengthUnit=m  TranslationStandardAxis=-X  TranslationCartesianOffset=[0 0 0]  TranslationROffset=0  TranslationROffsetUnits=m  TranslationZOffset=0  TranslationZOffsetUnits=m  TranslationThetaOffset=0  TranslationThetaOffsetUnits=deg  RotationMethod=None  RotationAngleUnits=deg  RotationStandardAxis=+Z  RotationAngle=0  RotationArbitraryAxis=[0 0 1]  FollAlignAxisA=+X  BaseAlignAxisA=+Y  FollAlignAxisB=+Y  BaseAlignAxisB=+Z  RotationSequenceAxes=FollowerAxes  RotationSequence=XYX  RotationSequenceAngles=[0 0 0]  RotationSequenceAnglesUnits=deg  RotationMatrix=[1 0 0; 0 1 0; 0 0 1]
  Right Crank Transform : sm_lib/Frames and Transforms/Rigid Transform  TranslationMethod=StandardAxis  TranslationStandardOffset=D/2  TranslationLengthUnit=m  TranslationStandardAxis=+X  TranslationCartesianOffset=[0 0 0]  TranslationROffset=0  TranslationROffsetUnits=m  TranslationZOffset=0  TranslationZOffsetUnits=m  TranslationThetaOffset=0  TranslationThetaOffsetUnits=deg  RotationMethod=None  RotationAngleUnits=deg  RotationStandardAxis=+Z  RotationAngle=0  RotationArbitraryAxis=[0 0 1]  FollAlignAxisA=+X  BaseAlignAxisA=+Y  FollAlignAxisB=+Y  BaseAlignAxisB=+Z  RotationSequenceAxes=FollowerAxes  RotationSequence=XYX  RotationSequenceAngles=[0 0 0]  RotationSequenceAnglesUnits=deg  RotationMatrix=[1 0 0; 0 1 0; 0 0 1]
  L : PMIOPort  Side=Left
  R : PMIOPort  Port=2  Side=Right
  connections:
  Left Crank Transform/RConn1 -- L/RConn1
  Left Crank Transform/LConn1 -- Right Crank Transform/LConn1 -- Crank/RConn1
  Right Crank Transform/RConn1 -- R/RConn1

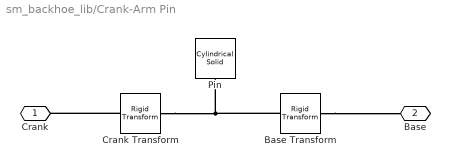
== system sm_backhoe_lib/Crank-Arm Pin ==
  Base Transform : sm_lib/Frames and Transforms/Rigid Transform  TranslationMethod=StandardAxis  TranslationStandardOffset=L/2  TranslationLengthUnit=m  TranslationStandardAxis=-Z  TranslationCartesianOffset=[0 0 0]  TranslationROffset=0  TranslationROffsetUnits=m  TranslationZOffset=0  TranslationZOffsetUnits=m  TranslationThetaOffset=0  TranslationThetaOffsetUnits=deg  RotationMethod=None  RotationAngleUnits=deg  RotationStandardAxis=+Z  RotationAngle=0  RotationArbitraryAxis=[0 0 1]  FollAlignAxisA=+X  BaseAlignAxisA=+Y  FollAlignAxisB=+Y  BaseAlignAxisB=+Z  RotationSequenceAxes=FollowerAxes  RotationSequence=XYX  RotationSequenceAngles=[0 0 0]  RotationSequenceAnglesUnits=deg  RotationMatrix=[1 0 0; 0 1 0; 0 0 1]
  Crank Transform : sm_lib/Frames and Transforms/Rigid Transform  TranslationMethod=StandardAxis  TranslationStandardOffset=L/2 - 0.65*T  TranslationLengthUnit=m  TranslationStandardAxis=+Z  TranslationCartesianOffset=[0 0 0]  TranslationROffset=0  TranslationROffsetUnits=m  TranslationZOffset=0  TranslationZOffsetUnits=m  TranslationThetaOffset=0  TranslationThetaOffsetUnits=deg  RotationMethod=None  RotationAngleUnits=deg  RotationStandardAxis=+Z  RotationAngle=0  RotationArbitraryAxis=[0 0 1]  FollAlignAxisA=+X  BaseAlignAxisA=+Y  FollAlignAxisB=+Y  BaseAlignAxisB=+Z  RotationSequenceAxes=FollowerAxes  RotationSequence=XYX  RotationSequenceAngles=[0 0 0]  RotationSequenceAnglesUnits=deg  RotationMatrix=[1 0 0; 0 1 0; 0 0 1]
  Pin : sm_lib/Body Elements/Cylindrical Solid  GraphicAmbientColor=[0.15 0.15 0.15 1.0]  BasedOnType=Density  CenterOfMass=[0 0 0]  CenterOfMassUnits=m  GraphicDiffuseColor=color  CylinderLength=L  CylinderLengthUnits=m  CylinderRadius=R  CylinderRadiusUnits=m  Density=rho  DensityUnits=kg/(m^3)  DoExposeReferenceFrame=on  GraphicEmissiveColor=[0.0 0.0 0.0 1.0]  ExportEntireGeometry=off  SerializedFrames=<Frames/>  MarkerShape=Sphere  MarkerSize=10  GraphicType=FromGeometry  InertiaType=CalculateFromGeometry  Mass=1  MassUnits=kg  MomentsOfInertia=[1 1 1]  MomentsOfInertiaUnits=kg*m^2  GraphicOpacity=1.0  ProductsOfInertia=[0 0 0]  ProductsOfInertiaUnits=kg*m^2  GraphicShininess=75  GraphicSpecularColor=[0.5 0.5 0.5 1.0]  GraphicVisPropType=SimpleVisualProperties
  Crank : PMIOPort  Side=Left
  Base : PMIOPort  Port=2  Side=Right
  connections:
  Crank Transform/RConn1 -- Crank/RConn1
  Crank Transform/LConn1 -- Base Transform/LConn1 -- Pin/RConn1
  Base Transform/RConn1 -- Base/RConn1

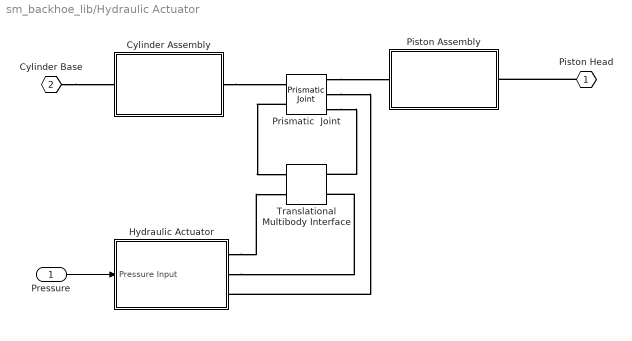
== system sm_backhoe_lib/Hydraulic Actuator ==
  Pressure : Inport
  Cylinder Assembly : Subsystem
  Hydraulic Actuator : Subsystem  VariantControl=var_hyd
  Piston Assembly : Subsystem
  Prismatic  Joint : sm_lib/Joints/Prismatic Joint  JointMode=Normal  SenseConstraintForce=off  SenseConstraintForceX=off  SenseConstraintForceY=off  SenseConstraintForceZ=off  SenseConstraintTorque=off  SenseConstraintTorqueX=off  SenseConstraintTorqueY=off  SenseConstraintTorqueZ=off  SenseTotalForce=off  SenseTotalForceX=off  SenseTotalForceY=off  SenseTotalForceZ=off  SenseTotalTorque=off  SenseTotalTorqueX=off  SenseTotalTorqueY=off  SenseTotalTorqueZ=off  CompositeWrenchDir=FollowerOnBase  CompositeWrenchFrame=BaseFrame  EquilibriumPosition=0  EquilibriumPositionUnits=m  SpringStiffness=0  SpringStiffnessUnits=N/m  DampingCoefficient=0  DampingCoefficientUnits=N/(m/s)  TorqueActuationMode=InputTorque  MotionActuationMode=ComputedMotion  SensePosition=on  SenseVelocity=on  SenseAcceleration=off  SenseTorqueForce=off  SenseLowerLimitTorqueForce=off  SenseUpperLimitTorqueForce=off  LowerLimitSpecify=off  LowerLimitBound=-1  LowerLimitBoundUnits=m  LowerLimitStiffness=1e6  LowerLimitStiffnessUnits=N/m  LowerLimitDamping=1e3  LowerLimitDampingUnits=N/(m/s)  LowerLimitTransitionRegionWidth=1e-4  LowerLimitTransitionRegionWidthUnits=m  UpperLimitSpecify=off  UpperLimitBound=1  UpperLimitBoundUnits=m  UpperLimitStiffness=1e6  UpperLimitStiffnessUnits=N/m  UpperLimitDamping=1e3  UpperLimitDampingUnits=N/(m/s)  UpperLimitTransitionRegionWidth=1e-4  UpperLimitTransitionRegionWidthUnits=m  PositionTargetSpecify=off  PositionTargetPriority=Low  PositionTargetValue=0  PositionTargetValueUnits=m  VelocityTargetSpecify=off  VelocityTargetPriority=High  VelocityTargetValue=0  VelocityTargetValueUnits=m/s
  Translational Multibody Interface : fl_lib/Mechanical/Multibody Interfaces/Translational Multibody Interface
      settings: SourceProductBaseCode=SS
  Piston Head : PMIOPort  Side=Right
  Cylinder Base : PMIOPort  Port=2  Side=Left
  wires:
  Pressure/1 -> Hydraulic Actuator/1(Pressure Input)
  connections:
  Cylinder Base/RConn1 -- Cylinder Assembly/RConn1
  Cylinder Assembly/LConn1 -- Prismatic  Joint/LConn1
  Prismatic  Joint/RConn1 -- Piston Assembly/LConn1
  Piston Head/RConn1 -- Piston Assembly/RConn1
  Hydraulic Actuator/RConn1 -- Translational Multibody Interface/LConn2
  Prismatic  Joint/LConn2 -- Translational Multibody Interface/LConn1
  Hydraulic Actuator/RConn2 -- Translational Multibody Interface/RConn2
  Prismatic  Joint/RConn3 -- Translational Multibody Interface/RConn1
  Prismatic  Joint/RConn2 -- Hydraulic Actuator/RConn3

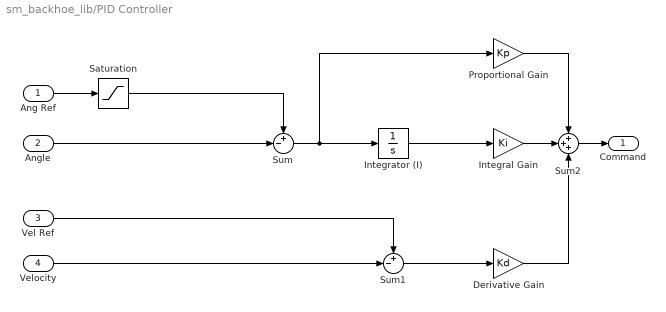
== system sm_backhoe_lib/PID Controller ==
  Ang Ref : Inport
  Angle : Inport  Port=2
  Vel Ref : Inport  Port=3
  Velocity : Inport  Port=4
  Derivative Gain : Gain  Gain=Kd
  Integral Gain : Gain  Gain=Ki
  Integrator (I) : Integrator
  Proportional Gain : Gain  Gain=Kp
  Saturation : Saturate  UpperLimit=upperLim  LowerLimit=lowerLim
  Sum : Sum  Inputs=+-|
  Sum1 : Sum  Inputs=+-|
  Sum2 : Sum  Inputs=+++
  Command : Outport  VectorParamsAs1DForOutWhenUnconnected=off
  wires:
  Vel Ref/1 -> Sum1/1
  Saturation/1 -> Sum/1
  Velocity/1 -> Sum1/2
  Angle/1 -> Sum/2
  Ang Ref/1 -> Saturation/1
  Sum2/1 -> Command/1
  Integrator (I)/1 -> Integral Gain/1
  Proportional Gain/1 -> Sum2/1
  Integral Gain/1 -> Sum2/2
  Sum/1 -> Integrator (I)/1, Proportional Gain/1
  Sum1/1 -> Derivative Gain/1
  Derivative Gain/1 -> Sum2/3

== system sm_backhoe_lib/Signal Generator ==
  Integrator : Integrator  InitialCondition=P(1)
  Repeating Sequence Interpolated2 : simulink/Sources/Repeating Sequence Interpolated  OutValues=V  TimeValues=Tv  LookUpMeth=Interpolation-Use End Values  tsamp=0.1  OutMin=[]  OutMax=[]  OutDataTypeStr=double  OutputDataTypeScalingMode=double  OutDataType=fixdt(0,8)  OutScaling=2^-10
  p : Outport  VectorParamsAs1DForOutWhenUnconnected=off
  v : Outport  Port=2  VectorParamsAs1DForOutWhenUnconnected=off
  wires:
  Integrator/1 -> p/1
  Repeating Sequence Interpolated2/1 -> Integrator/1, v/1

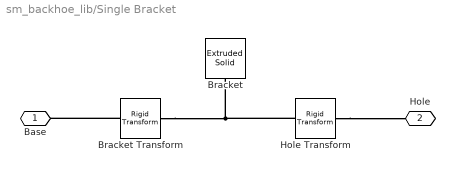
== system sm_backhoe_lib/Single Bracket ==
  Bracket : sm_lib/Body Elements/Extruded Solid  GraphicAmbientColor=[0.15 0.15 0.15 1.0]  BasedOnType=Density  CenterOfMass=[0 0 0]  CenterOfMassUnits=m  GraphicDiffuseColor=bracketColor  ExportConvexHullGeometry=off  ExtrusionCrossSection=bracketPoints  ExtrusionCrossSectionUnits=m  Density=rho  DensityUnits=kg/(m^3)  DoExposeReferenceFrame=on  GraphicEmissiveColor=[0.0 0.0 0.0 1.0]  ExportEntireGeometry=off  ExtrusionLength=Tbracket  ExtrusionLengthUnits=m  ExtrusionType=General  SerializedFrames=<Frames/>  MarkerShape=Sphere  MarkerSize=10  GraphicType=FromGeometry  InertiaType=CalculateFromGeometry  Mass=1  MassUnits=kg  MomentsOfInertia=[1 1 1]  MomentsOfInertiaUnits=kg*m^2  PolygonNumSides=3  GraphicOpacity=1.0  PolygonOuterRadius=1  PolygonOuterRadiusUnits=m  ProductsOfInertia=[0 0 0]  ProductsOfInertiaUnits=kg*m^2  GraphicShininess=75  GraphicSpecularColor=[0.5 0.5 0.5 1.0]  GraphicVisPropType=SimpleVisualProperties
  Bracket Transform : sm_lib/Frames and Transforms/Rigid Transform  TranslationMethod=None  TranslationStandardOffset=0  TranslationLengthUnit=m  TranslationStandardAxis=-Y  TranslationCartesianOffset=[0 0 0]  TranslationROffset=0  TranslationROffsetUnits=m  TranslationZOffset=0  TranslationZOffsetUnits=m  TranslationThetaOffset=0  TranslationThetaOffsetUnits=deg  RotationMethod=AlignedAxes  RotationAngleUnits=deg  RotationStandardAxis=+X  RotationAngle=90  RotationArbitraryAxis=[0 0 1]  FollAlignAxisA=+X  BaseAlignAxisA=+X  FollAlignAxisB=+Y  BaseAlignAxisB=+Z  RotationSequenceAxes=FollowerAxes  RotationSequence=XYX  RotationSequenceAngles=[0 0 0]  RotationSequenceAnglesUnits=deg  RotationMatrix=[1 0 0; 0 1 0; 0 0 1]
  Hole Transform : sm_lib/Frames and Transforms/Rigid Transform  TranslationMethod=StandardAxis  TranslationStandardOffset=Hhole  TranslationLengthUnit=m  TranslationStandardAxis=+Y  TranslationCartesianOffset=[0 0 0]  TranslationROffset=0  TranslationROffsetUnits=m  TranslationZOffset=0  TranslationZOffsetUnits=m  TranslationThetaOffset=0  TranslationThetaOffsetUnits=deg  RotationMethod=None  RotationAngleUnits=deg  RotationStandardAxis=+X  RotationAngle=90  RotationArbitraryAxis=[0 0 1]  FollAlignAxisA=+X  BaseAlignAxisA=+X  FollAlignAxisB=+Y  BaseAlignAxisB=+Z  RotationSequenceAxes=FollowerAxes  RotationSequence=XYX  RotationSequenceAngles=[0 0 0]  RotationSequenceAnglesUnits=deg  RotationMatrix=[1 0 0; 0 1 0; 0 0 1]
  Base : PMIOPort  Side=Left
  Hole : PMIOPort  Port=2  Side=Right
  connections:
  Hole Transform/LConn1 -- Bracket Transform/RConn1 -- Bracket/RConn1
  Hole Transform/RConn1 -- Hole/RConn1
  Bracket Transform/LConn1 -- Base/RConn1
